simulink model "DistributedEstimationFormation"  (R2022b)
settings: Solver=VariableStepAuto  StartTime=0.0  StopTime=params.T  RelTol=1e-3
undefined symbols (not defined in the file or in its folder): dfc_opnash, formation, graph, initial, model, params
settings Model: Creator=NTU  LastModifiedBy=NTU
settings DataIOCC: SaveState=on

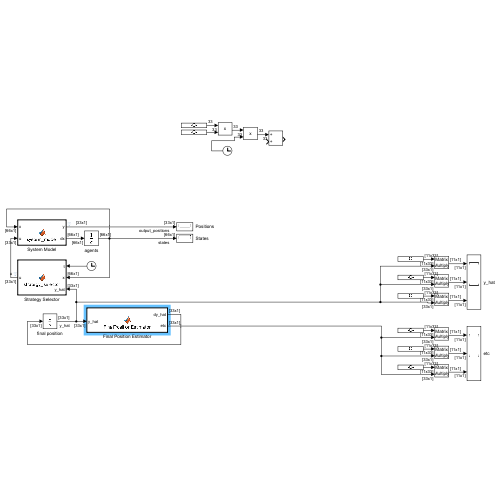
[thumbnail: Simulink's stored preview of the top-level diagram]
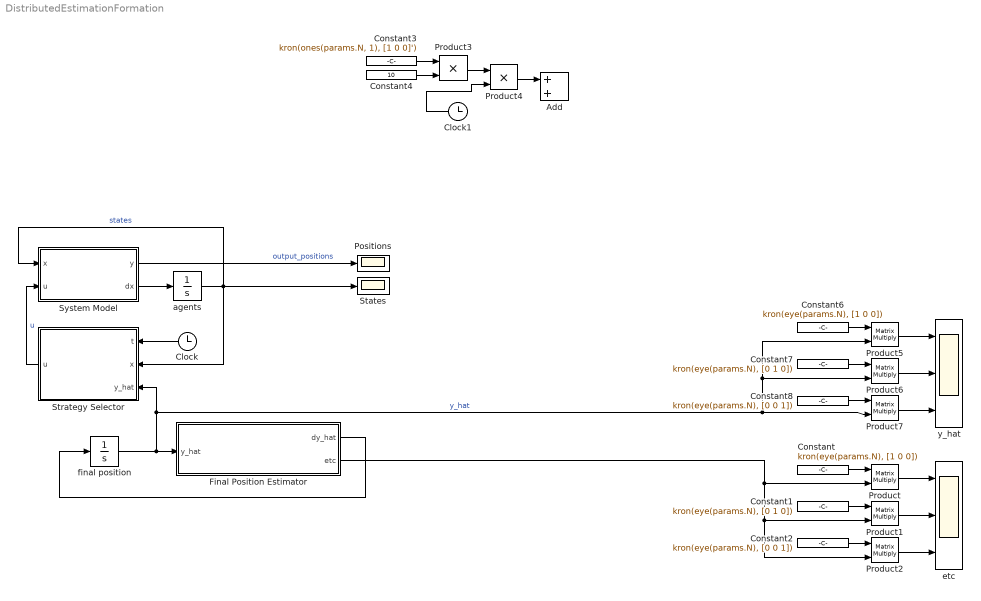
== system DistributedEstimationFormation ==
  Add : Sum
  Clock : Clock
  Clock1 : Clock
  Constant : Constant  Value=kron(eye(params.N), [1 0 0])
  Constant1 : Constant  Value=kron(eye(params.N), [0 1 0])
  Constant2 : Constant  Value=kron(eye(params.N), [0 0 1])
  Constant3 : Constant  Value=kron(ones(params.N, 1), [1 0 0]')
  Constant4 : Constant  Value=10
  Constant6 : Constant  Value=kron(eye(params.N), [1 0 0])
  Constant7 : Constant  Value=kron(eye(params.N), [0 1 0])
  Constant8 : Constant  Value=kron(eye(params.N), [0 0 1])
  Final Position Estimator : MATLAB Function  TreatAsAtomicUnit=on
  Positions : Scope
  Product{,1..2,5..7} (6 alike) : Product  Multiplication=Matrix(*)
  Product3 : Product
  Product4 : Product
  States : Scope
  Strategy Selector : MATLAB Function  TreatAsAtomicUnit=on
  System Model : MATLAB Function  TreatAsAtomicUnit=on
  agents : Integrator  InitialCondition=initial.state  ContinuousStateAttributes='x'
  etc : Scope  NumInputPorts=3
  final position : Integrator  InitialCondition=initial.pos  ContinuousStateAttributes='y_hat'
  y_hat : Scope  NumInputPorts=3
  wires:
  System Model/2(dx) -> agents/1
  agents/1 -> Strategy Selector/2(x), System Model/1(x), States/1  "states"
  Clock/1 -> Strategy Selector/1(t)
  System Model/1(y) -> Positions/1  "output_positions"
  final position/1 -> Product7/2, Product5/2, Product6/2, Strategy Selector/3(y_hat), Final Position Estimator/1(y_hat)  "y_hat"
  Final Position Estimator/1(dy_hat) -> final position/1
  Constant/1 -> Product/1
  Product/1 -> etc/1
  Product1/1 -> etc/2
  Product2/1 -> etc/3
  Constant1/1 -> Product1/1
  Constant2/1 -> Product2/1
  Final Position Estimator/2(etc) -> Product2/2, Product1/2, Product/2
  Constant3/1 -> Product3/1
  Constant4/1 -> Product3/2
  Product3/1 -> Product4/1
  Clock1/1 -> Product4/2
  Product4/1 -> Add/1
  Constant8/1 -> Product7/1
  Product6/1 -> y_hat/2
  Product7/1 -> y_hat/3
  Product5/1 -> y_hat/1
  Constant6/1 -> Product5/1
  Constant7/1 -> Product6/1
  Strategy Selector/1(u) -> System Model/2(u)  "u"

== matlab function DistributedEstimationFormation/Strategy Selector ==
  data: t input; x input; y_hat input; u output; params parameter; formation parameter; model parameter; graph parameter; dfc_opnash parameter
function u = strategy_selector(t, x, y_hat, params, formation, model, graph, dfc_opnash)
    % u = open_loop_nash(t, x, params, initial, model, graph, dfc_opnash);
    u = distributed_open_loop_nash(t, x, y_hat, params, formation, model, graph, dfc_opnash);
end

== matlab function DistributedEstimationFormation/System Model ==
  data: y output; x input; u input; dx output; params parameter; model parameter
function [y, dx] = system_model(x, u, params, model)
    n = params.n;
    m = params.m;
    p = params.p;
   
    dx = zeros(params.N * params.n, 1);
    y = zeros(params.N * params.m, 1);
    for i = 1:params.N
        [dx((i-1)*n+1 : i*n), y((i-1)*m+1 : i*m)] = ...
            agent_model(x((i-1)*n+1 : i*n), u((i-1)*p+1 : i*p), model);
    end
end

== matlab function DistributedEstimationFormation/Final Position Estimator ==
  settings: updateMethod=CONTINUOUS  sampleTime=0.01
  data: y_hat input; params parameter; initial parameter; model parameter; graph parameter; dfc_opnash parameter; formation parameter; dy_hat output; etc output
function [dy_hat, etc]  = FinalPositionEstimator(y_hat, params, initial, model, graph, dfc_opnash, formation)
    [dy_hat, etc] = final_position_estimator(y_hat, params, initial, model, graph, formation, dfc_opnash);
end
